simulink model "Module1QuizModel"  (R2026a)
settings: Solver=VariableStepAuto  StopTime=7200
libraries: fl_lib x4, batt_lib x2, simulink x2, nesl_utility x1
settings Model: Creator=sturton  LastModifiedBy=User
settings SimscapeCC: SimscapeNominalValues="[{\"value\":\"1\",\"unit\":\"A\"},{\"value\":\"1\",\"unit\":\"bar\"},{\"value\":\"1\",\"unit\":\"cm^2\"},{\"value\":\"1\",\"unit\":\"cm^3/s\"},{\"value\":\"1\",\"unit\":\"kJ/kg\"},{\"value\":\"1\",\"unit\":\"kW\"},{\"value\":\"1\",\"unit\":\"l\"},{\"value\":\"1\",\"unit\":\"N\"},{\"value\":\"1\",\"unit\":\"N*m\"},{\"value\":\"1\",\"unit\":\"V\"}]"  SimscapeLogType=none  SimscapeLogDataHistory=5000.0

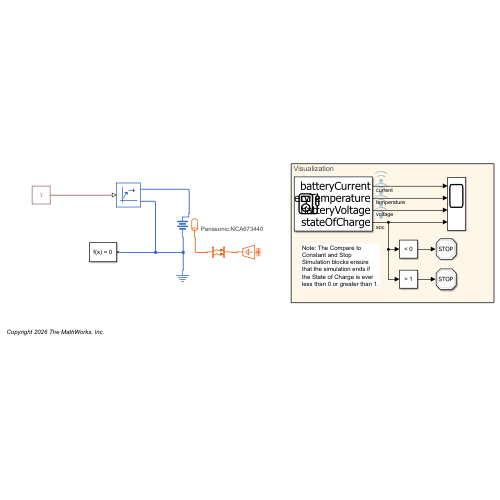
[thumbnail: Simulink's stored preview of the top-level diagram]
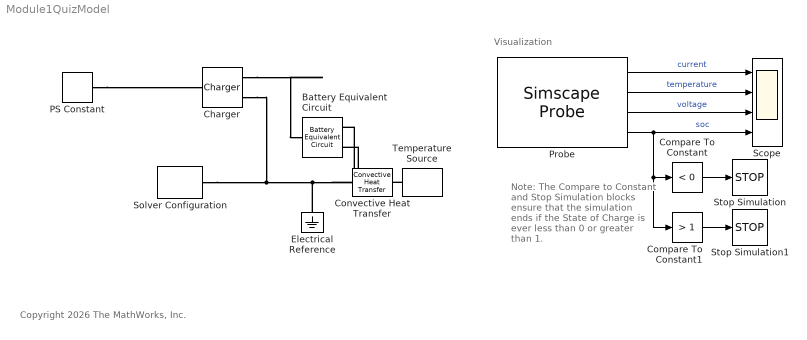
== system Module1QuizModel ==
  note: Note: The Compare to Constant and Stop Simulation blocks ensure that the simulation ends if the State of Charge is ever less than 0 or greater than 1.
  note: Visualization
  note: Copyright 2026 The MathWorks, Inc.
  Battery Equivalent Circuit : batt_lib/Cells/Battery Equivalent Circuit  PartSpecification="{\"CollectionId\":\"MW.SimscapeBattery\",\"CollectionVersion\":\"1.0.0\",\"DatasetId\":\"Panasonic|NCA673440|simscape.battery.batteryEquivalentCircuit\",\"DisplayName\":\"Panasonic:NCA673440\"}"  BatteryCapacity=1.236 % Datasheet derived hr*A  ThermalModel=simscape.battery.enum.cells.BatteryThermalModel.LumpedThermalMass  ExtrapolationMethod=simscape.enum.extrapolation.linear  SOCBreakpoints=[0 0.01 0.02 0.03 0.04 0.05 0.06 0.07 0.08 0.09 0.1 0.11 0.12 0.13 0.14 0.15 0.16 0.17 0.18 0.19 0.2 0.21 0.22 0.23 0.24 0.25 0.26 0.27 0.28 0.29 0.3 0.31 0.32 0.33 0.34 0.35 0.36 0.37 0.38 0.39 0.4 0.41 0.42 0.43 0.44 0.45 0.46 0.47 0.48 0.49 0.5 0.51 0.52 0.53 0.54 0.55 0.56 0.57 0.58 0.59 0.6 0.61 0.62 0.63 0.64 0.65 0.66 0.67 0.68 0.69 0.7 0.71 0.72 0.73 0.74 0.75 0.76 0.77 0.78 0.79 0.8 0.81 0.82 0.83 0.84 0.85 0.86 0.87 0.88 0.89 0.9 0.91 0.92 0.93 0.94 0.95 0.96 0.97 0.98 0.99 1] % Datasheet derived  TemperatureBreakpoints=[-20 -10 0 25 40] % Datasheet derived degC  OpenCircuitVoltage=[2.81282 2.92952 3.02616 3.09882 3.15595 3.19736 3.23687 3.2696 3.29224 3.3165 3.33606 3.35376 3.37201 3.38673 3.40034 3.412 3.42329 3.4339 3.44451 3.45615 3.466 3.4726 3.47919 3.48579 3.49239 3.49904 3.50604 3.51305 3.52005 3.52703 3.53325 3.53921 3.54518 3.55115 3.55712 3.56323 3.5696 3.57596 3.58233 3.58876 3.59531 3.60186 3.60839 3.61485 3.62133 3.62799 3.63464 3.64129 3.64862 3.65637 3.6643 3.67241 3.68051 3.68861 3.69647 3.70506 3.71368 3.7223 3.731 3.74039 3.74966 3.75893 3.76819 3.77737 3.78644 3.79552 3.80425 3.81234 3.82043 3.82859 3.83695 3.84539 3.85383 3.86227 3.87071 3.87916 3.8876 3.89604 3.90651 3.91746 3.92861 3.94006 3.95152 3.96297 3.97442 3.98588 3.99733 4.0089 4.02025 4.03129 4.04215 4.0529 4.06366 4.07442 4.0852 4.09635 4.1089 4.1233 4.13483 4.15326 4.13871] % Datasheet derived V  OpenCircuitVoltageThermal=[2.81282 2.81282 2.81282 2.81282 2.81282;2.92952 2.92952 2.92952 2.92952 2.92952;3.02616 3.02616 3.02616 3.02616 3.02616;3.09882 3.09882 3.09882 3.09882 3.09882;3.15595 3.15595 3.15595 3.15595 3.15595;3.19736 3.19736 3.19736 3.19736 3.19736;3.23687 3.23687 3.23687 3.23687 3.23687;3.2696 3.2696 3.2696 3.2696 3.2696;3.29224 3.29224 3.29224 3.29224 3.29224;3.3165 3.3165 3.3165 3.3165 3.3165;3.33606 3.33606 3.33606 3.33606 3.33606;3.35376 3.35376 3.35376 3.35376 3.35376;3.37201 3.37201 3.37201 3.37201 3.37201;3.38673 3.38673 3.38673 3.38673 3.38673;3.40034 3.40034 3.40034 3.40034 3.40034;3.412 3.412 3.412 3.412 3.412;3.42329 3.42329 3.42329 3.42329 3.42329;3.4339 3.4339 3.4339 3.4339 3.4339;3.44451 3.44451 3.44451 3.44451 3.44451;3.45615 3.45615 3.45615 3.45615 3.45615;3.466 3.466 3.466 3.466 3.466;3.4726 3.4726 3.4726 3.4726 3.4726;3.47919 3.47919 3.47919 3.47919 3.47919;3.48579 3.48579 3.48579 3.48579 3.48579;3.49239 3.49239 3.49239 3.49239 3.49239;3.49904 3.49904 3.49904 3.49904 3.49904;3.50604 3.50604 3.50604 3.50604 3.50604;3.51305 3.51305 3.51305 3.51305 3.51305;3.52005 3.52005 3.52005 3.52005 3.52005;3.52703 3.52703 3.52703 3.52703 3.52703;3.53325 3.53325 3.53325 3.53325 3.53325;3.53921 3.53921 3.53921 3.53921 3.53921;3.54518 3.54518 3.54518 3.54518 3.54518;3.55115 3.55115 3.55115 3.55115 3.55115;3.55712 3.55712 3.55712 3.55712 3.55712;3.56323 3.56323 3.56323 3.56323 3.56323;3.5696 3.5696 3.5696 3.5696 3.5696;3.57596 3.57596 3.57596 3.57596 3.57596;3.58233 3.58233 3.58233 3.58233 3.58233;3.58876 3.58876 3.58876 3.58876 3.58876;3.59531 3.59531 3.59531 3.59531 3.59531;3.60186 3.60186 3.60186 3.60186 3.60186;3.60839 3.60839 3.60839 3.60839 3.60839;3.61485 3.61485 3.61485 3.61485 3.61485;3.62133 3.62133 3.62133 3.62133 3.62133;3.62799 3.62799 3.62799 3.62799 3.62799;3.63464 3.63464 3.63464 3.63464 3.63464;3.64129 3.64129 3.64129 3.64129 3.64129;3.64862 3.64862 3.64862 3.64862 3.64862;3.65637 3.65637 3.65637 3.65637 3.65637;3.6643 3.6643 3.6643 3.6643 3.6643;3.67241 3.67241 3.67241 3.67241 3.67241;3.68051 3.68051 3.68051 3.68051 3.68051;3.68861 3.68861 3.68861 3.68861 3.68861;3.69647 3.69647 3.69647 3.69647 3.69647;3.70506 3.70506 3.70506 3.70506 3.70506;3.71368 3.71368 3.71368 3.71368 3.71368;3.7223 3.7223 3.7223 3.7223 3.7223;3.731 3.731 3.731 3.731 3.731;3.74039 3.74039 3.74039 3.74039 3.74039;3.74966 3.74966 3.74966 3.74966 3.74966;3.75893 3.75893 3.75893 3.75893 3.75893;3.76819 3.76819 3.76819 3.76819 3.76819;3.77737 3.77737 3.77737 3.77737 3.77737;3.78644 3.78644 3.78644 3.78644 3.78644;3.79552 3.79552 3.79552 3.79552 3.79552;3.80425 3.80425 3.80425 3.80425 3.80425;3.81234 3.81234 3.81234 3.81234 3.81234;3.82043 3.82043 3.82043 3.82043 3.82043;3.82859 3.82859 3.82859 3.82859 3.82859;3.83695 3.83695 3.83695 3.83695 3.83695;3.84539 3.84539 3.84539 3.84539 3.84539;3.85383 3.85383 3.85383 3.85383 3.85383;3.86227 3.86227 3.86227 3.86227 3.86227;3.87071 3.87071 3.87071 3.87071 3.87071;3.87916 3.87916 3.87916 3.87916 3.87916;3.8876 3.8876 3.8876 3.8876 3.8876;3.89604 3.89604 3.89604 3.89604 3.89604;3.90651 3.90651 3.90651 3.90651 3.90651;3.91746 3.91746 3.91746 3.91746 3.91746;3.92861 3.92861 3.92861 3.92861 3.92861;3.94006 3.94006 3.94006 3.94006 3.94006;3.95152 3.95152 3.95152 3.95152 3.95152;3.96297 3.96297 3.96297 3.96297 3.96297;3.97442 3.97442 3.97442 3.97442 3.97442;3.98588 3.98588 3.98588 3.98588 3.98588;3.99733 3.99733 3.99733 3.99733 3.99733;4.0089 4.0089 4.0089 4.0089 4.0089;4.02025 4.02025 4.02025 4.02025 4.02025;4.03129 4.03129 4.03129 4.03129 4.03129;4.04215 4.04215 4.04215 4.04215 4.04215;4.0529 4.0529 4.0529 4.0529 4.0529;4.06366 4.06366 4.06366 4.06366 4.06366;4.07442 4.07442 4.07442 4.07442 4.07442;4.0852 4.0852 4.0852 4.0852 4.0852;4.09635 4.09635 4.09635 4.09635 4.09635;4.1089 4.1089 4.1089 4.1089 4.1089;4.1233 4.1233 4.1233 4.1233 4.1233;4.13483 4.13483 4.13483 4.13483 4.13483;4.15326 4.15326 4.15326 4.15326 4.15326;4.13871 4.13871 4.13871 4.13871 4.13871] % Datasheet derived V  VoltageRange=[2.475 Inf] % Datasheet derived V  HysteresisModel=simscape.battery.enum.cells.HysteresisModel.none  MaximumHysteresisVoltage=[0, 0, 0, 0, 0, 0, 0] % Parameter not set V  InstantaneousHysteresisVoltage=[0, 0, 0, 0, 0, 0, 0] % Parameter not set V  HysteresisRate=0.1 % Parameter not set  MaximumHysteresisVoltageThermal=[0, 0, 0; 0, 0, 0; 0, 0, 0; 0, 0, 0; 0, 0, 0; 0, 0, 0; 0, 0, 0] % Parameter not set V  InstantaneousHysteresisVoltageThermal=[0, 0, 0; 0, 0, 0; 0, 0, 0; 0, 0, 0; 0, 0, 0; 0, 0, 0; 0, 0, 0] % Parameter not set V  HysteresisRateThermal=0.1 % Parameter not set  ResistanceSOCBreakpoints=[0 0.01 0.02 0.03 0.04 0.05 0.06 0.07 0.08 0.09 0.1 0.11 0.12 0.13 0.14 0.15 0.16 0.17 0.18 0.19 0.2 0.21 0.22 0.23 0.24 0.25 0.26 0.27 0.28 0.29 0.3 0.31 0.32 0.33 0.34 0.35 0.36 0.37 0.38 0.39 0.4 0.41 0.42 0.43 0.44 0.45 0.46 0.47 0.48 0.49 0.5 0.51 0.52 0.53 0.54 0.55 0.56 0.57 0.58 0.59 0.6 0.61 0.62 0.63 0.64 0.65 0.66 0.67 0.68 0.69 0.7 0.71 0.72 0.73 0.74 0.75 0.76 0.77 0.78 0.79 0.8 0.81 0.82 0.83 0.84 0.85 0.86 0.87 0.88 0.89 0.9 0.91 0.92 0.93 0.94 0.95 0.96 0.97 0.98 0.99 1] % Datasheet derived  ResistanceTemperatureBreakpoints=[-20 -10 0 25 40] % Datasheet derived degC  ResistanceCurrentBreakpoints=[-1, 0, 1] % Parameter not set A  CurrentDependence=simscape.battery.enum.cells.CurrentDependence.Disabled  R0=[0.1195 0.14734 0.16452 0.17097 0.16988 0.16446 0.16485 0.16445 0.16084 0.15998 0.15922 0.15784 0.1574 0.1565 0.15518 0.15284 0.15055 0.14837 0.14619 0.14574 0.14532 0.1435 0.14169 0.13987 0.13805 0.13632 0.13519 0.13407 0.13294 0.1318 0.13054 0.1292 0.12787 0.12654 0.1252 0.12412 0.12346 0.1228 0.12215 0.12145 0.12073 0.12001 0.11928 0.11852 0.11781 0.11738 0.11695 0.11652 0.11644 0.1166 0.11673 0.11683 0.11693 0.11703 0.11671 0.1163 0.11591 0.11551 0.11516 0.11517 0.11521 0.11524 0.11527 0.11514 0.11486 0.11457 0.11414 0.11345 0.11275 0.11209 0.11172 0.1115 0.11127 0.11105 0.11082 0.1106 0.11037 0.11014 0.11063 0.11131 0.11219 0.1136 0.115 0.11641 0.11781 0.11921 0.12062 0.12211 0.12357 0.1249 0.12592 0.12677 0.12761 0.12845 0.12929 0.13023 0.13186 0.13449 0.1303 0.12272 0.05007] % Datasheet derived Ohm  R0I=[.0117, .0085, .009; .011, .0085, .009; .0114, .0087, .0092; .0107, .0082, .0088; .0107, .0083, .0091; .0113, .0085, .0089; .0116, .0085, .0089] % Parameter not set Ohm  R0Thermal=[0.91507 0.64886 0.76779 0.1195 0.07217;0.91507 0.9802 1.05708 0.14734 0.05983;0.91507 0.95979 1.01635 0.16452 0.04254;0.91507 0.93938 0.97562 0.17097 0.05718;0.91507 0.91897 0.93489 0.16988 0.06137;0.91507 0.89855 0.89416 0.16446 0.07086;0.91507 0.87814 0.85343 0.16485 0.07883;0.91507 0.85773 0.8127 0.16445 0.09222;0.91507 0.83732 0.77197 0.16084 0.09721;0.91507 0.81691 0.73124 0.15998 0.10355;0.91507 0.7965 0.69051 0.15922 0.10881;0.91507 0.77608 0.64978 0.15784 0.11252;0.91507 0.75567 0.60905 0.1574 0.11668;0.90135 0.73526 0.56832 0.1565 0.11813;0.88763 0.71485 0.52759 0.15518 0.11951;0.87392 0.69444 0.48527 0.15284 0.11926;0.8602 0.67403 0.45861 0.15055 0.1187;0.84648 0.65361 0.43204 0.14837 0.11758;0.83276 0.6332 0.41039 0.14619 0.11645;0.81904 0.61279 0.39684 0.14574 0.11867;0.80533 0.59091 0.38181 0.14532 0.11977;0.79161 0.56633 0.36407 0.1435 0.11817;0.77789 0.54174 0.3476 0.14169 0.11656;0.76417 0.51715 0.33715 0.13987 0.11495;0.75045 0.49671 0.32669 0.13805 0.11335;0.73674 0.48301 0.31628 0.13632 0.11191;0.72302 0.4696 0.30882 0.13519 0.11096;0.7093 0.4562 0.30303 0.13407 0.11001;0.69558 0.4428 0.29723 0.13294 0.10905;0.68186 0.42937 0.29142 0.1318 0.10807;0.66815 0.41843 0.28497 0.13054 0.10646;0.65423 0.41062 0.28038 0.1292 0.10465;0.64032 0.40281 0.27663 0.12787 0.10283;0.6264 0.395 0.27288 0.12654 0.10101;0.61249 0.38719 0.26913 0.1252 0.09919;0.5987 0.3795 0.2655 0.12412 0.09826;0.58512 0.37203 0.26209 0.12346 0.0977;0.57153 0.36581 0.25916 0.1228 0.09714;0.55932 0.36186 0.25623 0.12215 0.09658;0.55177 0.35796 0.25335 0.12145 0.09608;0.54432 0.35417 0.25057 0.12073 0.09567;0.53687 0.35037 0.24779 0.12001 0.09527;0.5294 0.34656 0.24499 0.11928 0.09484;0.52187 0.34269 0.24214 0.11852 0.09436;0.51437 0.33884 0.2393 0.11781 0.0939;0.507 0.33512 0.23677 0.11738 0.09322;0.50125 0.33141 0.23475 0.11695 0.0919;0.49572 0.32777 0.23274 0.11652 0.09057;0.49076 0.3247 0.23129 0.11644 0.08981;0.48615 0.32199 0.23019 0.1166 0.0894;0.48169 0.31942 0.22925 0.11673 0.08914;0.47738 0.317 0.22844 0.11683 0.08902;0.47306 0.31457 0.22764 0.11693 0.0889;0.46874 0.31215 0.22683 0.11703 0.08879;0.46462 0.30952 0.22582 0.11671 0.08846;0.46133 0.3075 0.22542 0.1163 0.08795;0.45807 0.30632 0.22505 0.11591 0.08735;0.4548 0.3054 0.22468 0.11551 0.08676;0.4516 0.30454 0.22428 0.11516 0.08623;0.44899 0.30426 0.22355 0.11517 0.08628;0.44626 0.30388 0.22271 0.11521 0.08622;0.44354 0.3035 0.22188 0.11524 0.08617;0.44082 0.30312 0.22104 0.11527 0.08611;0.43851 0.30265 0.22013 0.11514 0.08598;0.4385 0.30212 0.21913 0.11486 0.08576;0.4385 0.30158 0.21814 0.11457 0.08555;0.4382 0.30094 0.21686 0.11414 0.08505;0.43737 0.30006 0.21504 0.11345 0.08401;0.43654 0.29918 0.21322 0.11275 0.08322;0.43576 0.29836 0.21146 0.11209 0.08264;0.43516 0.2977 0.21187 0.11172 0.08223;0.43462 0.29712 0.21246 0.1115 0.08189;0.43513 0.29653 0.21305 0.11127 0.08154;0.43636 0.29594 0.21363 0.11105 0.0812;0.43759 0.29536 0.21422 0.11082 0.08086;0.43882 0.29583 0.21481 0.1106 0.08051;0.44004 0.29808 0.21539 0.11037 0.08017;0.44127 0.30032 0.21598 0.11014 0.07983;0.44419 0.30425 0.21826 0.11063 0.08056;0.4475 0.30858 0.22093 0.11131 0.08006;0.45099 0.31308 0.22434 0.11219 0.07972;0.45473 0.31784 0.22962 0.1136 0.07964;0.46234 0.32313 0.2349 0.115 0.07955;0.47176 0.33193 0.24018 0.11641 0.07947;0.48119 0.34073 0.24546 0.11781 0.07938;0.49061 0.34953 0.25074 0.11921 0.0793;0.50004 0.35833 0.25602 0.12062 0.07955;0.50956 0.36723 0.2645 0.12211 0.0805;0.5224 0.37673 0.27312 0.12357 0.08126;0.54766 0.39209 0.28148 0.1249 0.08177;0.57277 0.4073 0.2897 0.12592 0.08213;0.60249 0.42242 0.29782 0.12677 0.0824;0.63849 0.43753 0.30705 0.12761 0.08267;0.67449 0.45424 0.31684 0.12845 0.08292;0.71052 0.47435 0.32664 0.12929 0.08317;0.7543 0.49476 0.33675 0.13023 0.08373;0.79949 0.51481 0.34571 0.13186 0.08544;0.84623 0.53557 0.355 0.13449 0.08871;0.86284 0.54572 0.36189 0.1303 0.08803;0.87986 0.53749 0.35636 0.12272 0.08074;0.76995 0.47785 0.31756 0.05007 0.04597] % Datasheet derived Ohm  R0ThermalI=repmat([.0117, .0085, .009; .011, .0085, .009; .0114, .0087, .0092; .0107, .0082, .0088; .0107, .0083, .0091; .0113, .0085, .0089; .0116, .0085, .0089], 1, 1, 3) % Parameter not set Ohm  DischargeR0=[.0085, .0085, .0087, .0082, .0083, .0085, .0085] % Parameter not set Ohm  ChargeR0=[.0085, .0085, .0087, .0082, .0083, .0085, .0085] % Parameter not set Ohm  ChargeR0Thermal=[.0117, .0085, .009; .011, .0085, .009; .0114, .0087, .0092; .0107, .0082, .0088; .0107, .0083, .0091; .0113, .0085, .0089; .0116, .0085, .0089] % Parameter not set Ohm  DischargeR0Thermal=[.0117, .0085, .009; .011, .0085, .009; .0114, .0087, .0092; .0107, .0082, .0088; .0107, .0083, .0091; .0113, .0085, .0089; .0116, .0085, .0089] % Parameter not set Ohm  RCPairs=simscape.battery.enum.cells.RCPairs.noDynamics  R1=[.0029, .0024, .0026, .0016, .0023, .0018, .0017] % Parameter not set Ohm  Tau1=[36, 45, 105, 29, 77, 33, 39] % Parameter not set s  R2=[.0029, .0024, .0026, .0016, .0023, .0018, .0017] % Parameter not set Ohm  Tau2=[36, 45, 105, 29, 77, 33, 39] % Parameter not set s  R3=[.0029, .0024, .0026, .0016, .0023, .0018, .0017] % Parameter not set Ohm  Tau3=[36, 45, 105, 29, 77, 33, 39] % Parameter not set s  R1I=[.0109, .0029, .0013; .0069, .0024, .0012; .0047, .0026, .0013; .0034, .0016, .001; .0033, .0023, .0014; .0033, .0018, .0011; .0028, .0017, .0011] % Parameter not set Ohm  Tau1I=[20, 36, 39; 31, 45, 39; 109, 105, 61; 36, 29, 26; 59, 77, 67; 40, 33, 29; 25, 39, 33] % Parameter not set s  R2I=[.0109, .0029, .0013; .0069, .0024, .0012; .0047, .0026, .0013; .0034, .0016, .001; .0033, .0023, .0014; .0033, .0018, .0011; .0028, .0017, .0011] % Parameter not set Ohm  Tau2I=[20, 36, 39; 31, 45, 39; 109, 105, 61; 36, 29, 26; 59, 77, 67; 40, 33, 29; 25, 39, 33] % Parameter not set s  R3I=[.0109, .0029, .0013; .0069, .0024, .0012; .0047, .0026, .0013; .0034, .0016, .001; .0033, .0023, .0014; .0033, .0018, .0011; .0028, .0017, .0011] % Parameter not set Ohm  Tau3I=[20, 36, 39; 31, 45, 39; 109, 105, 61; 36, 29, 26; 59, 77, 67; 40, 33, 29; 25, 39, 33] % Parameter not set s  DischargeR1=[.0029, .0024, .0026, .0016, .0023, .0018, .0017] % Parameter not set Ohm  DischargeTau1=[36, 45, 105, 29, 77, 33, 39] % Parameter not set s  ChargeR1=[.0029, .0024, .0026, .0016, .0023, .0018, .0017] % Parameter not set Ohm  ChargeTau1=[36, 45, 105, 29, 77, 33, 39] % Parameter not set s  DischargeR2=[.0029, .0024, .0026, .0016, .0023, .0018, .0017] % Parameter not set Ohm  DischargeTau2=[36, 45, 105, 29, 77, 33, 39] % Parameter not set s  ChargeR2=[.0029, .0024, .0026, .0016, .0023, .0018, .0017] % Parameter not set Ohm  ChargeTau2=[36, 45, 105, 29, 77, 33, 39] % Parameter not set s  DischargeR3=[.0029, .0024, .0026, .0016, .0023, .0018, .0017] % Parameter not set Ohm  DischargeTau3=[36, 45, 105, 29, 77, 33, 39] % Parameter not set s  ChargeR3=[.0029, .0024, .0026, .0016, .0023, .0018, .0017] % Parameter not set Ohm  ChargeTau3=[36, 45, 105, 29, 77, 33, 39] % Parameter not set s  R1Thermal=[.0109, .0029, .0013; .0069, .0024, .0012; .0047, .0026, .0013; .0034, .0016, .001; .0033, .0023, .0014; .0033, .0018, .0011; .0028, .0017, .0011] % Parameter not set Ohm  Tau1Thermal=[20, 36, 39; 31, 45, 39; 109, 105, 61; 36, 29, 26; 59, 77, 67; 40, 33, 29; 25, 39, 33] % Parameter not set s  R2Thermal=[.0109, .0029, .0013; .0069, .0024, .0012; .0047, .0026, .0013; .0034, .0016, .001; .0033, .0023, .0014; .0033, .0018, .0011; .0028, .0017, .0011] % Parameter not set Ohm  Tau2Thermal=[20, 36, 39; 31, 45, 39; 109, 105, 61; 36, 29, 26; 59, 77, 67; 40, 33, 29; 25, 39, 33] % Parameter not set s  R3Thermal=[.0109, .0029, .0013; .0069, .0024, .0012; .0047, .0026, .0013; .0034, .0016, .001; .0033, .0023, .0014; .0033, .0018, .0011; .0028, .0017, .0011] % Parameter not set Ohm  Tau3Thermal=[20, 36, 39; 31, 45, 39; 109, 105, 61; 36, 29, 26; 59, 77, 67; 40, 33, 29; 25, 39, 33] % Parameter not set s  R1ThermalI=repmat([.0109, .0029, .0013; .0069, .0024, .0012; .0047, .0026, .0013; .0034, .0016, .001; .0033, .0023, .0014; .0033, .0018, .0011; .0028, .0017, .0011], 1, 1, 3) % Parameter not set Ohm  Tau1ThermalI=repmat([20, 36, 39; 31, 45, 39; 109, 105, 61; 36, 29, 26; 59, 77, 67; 40, 33, 29; 25, 39, 33], 1, 1, 3) % Parameter not set s  R2ThermalI=repmat([.0109, .0029, .0013; .0069, .0024, .0012; .0047, .0026, .0013; .0034, .0016, .001; .0033, .0023, .0014; .0033, .0018, .0011; .0028, .0017, .0011], 1, 1, 3) % Parameter not set Ohm  Tau2ThermalI=repmat([20, 36, 39; 31, 45, 39; 109, 105, 61; 36, 29, 26; 59, 77, 67; 40, 33, 29; 25, 39, 33], 1, 1, 3) % Parameter not set s  R3ThermalI=repmat([.0109, .0029, .0013; .0069, .0024, .0012; .0047, .0026, .0013; .0034, .0016, .001; .0033, .0023, .0014; .0033, .0018, .0011; .0028, .0017, .0011], 1, 1, 3) % Parameter not set Ohm  Tau3ThermalI=repmat([20, 36, 39; 31, 45, 39; 109, 105, 61; 36, 29, 26; 59, 77, 67; 40, 33, 29; 25, 39, 33], 1, 1, 3) % Parameter not set s  DischargeR1Thermal=[.0109, .0029, .0013; .0069, .0024, .0012; .0047, .0026, .0013; .0034, .0016, .001; .0033, .0023, .0014; .0033, .0018, .0011; .0028, .0017, .0011] % Parameter not set Ohm  DischargeTau1Thermal=[20, 36, 39; 31, 45, 39; 109, 105, 61; 36, 29, 26; 59, 77, 67; 40, 33, 29; 25, 39, 33] % Parameter not set s  ChargeR1Thermal=[.0109, .0029, .0013; .0069, .0024, .0012; .0047, .0026, .0013; .0034, .0016, .001; .0033, .0023, .0014; .0033, .0018, .0011; .0028, .0017, .0011] % Parameter not set Ohm  ChargeTau1Thermal=[20, 36, 39; 31, 45, 39; 109, 105, 61; 36, 29, 26; 59, 77, 67; 40, 33, 29; 25, 39, 33] % Parameter not set s  DischargeR2Thermal=[.0109, .0029, .0013; .0069, .0024, .0012; .0047, .0026, .0013; .0034, .0016, .001; .0033, .0023, .0014; .0033, .0018, .0011; .0028, .0017, .0011] % Parameter not set Ohm  DischargeTau2Thermal=[20, 36, 39; 31, 45, 39; 109, 105, 61; 36, 29, 26; 59, 77, 67; 40, 33, 29; 25, 39, 33] % Parameter not set s  ChargeR2Thermal=[.0109, .0029, .0013; .0069, .0024, .0012; .0047, .0026, .0013; .0034, .0016, .001; .0033, .0023, .0014; .0033, .0018, .0011; .0028, .0017, .0011] % Parameter not set Ohm  ChargeTau2Thermal=[20, 36, 39; 31, 45, 39; 109, 105, 61; 36, 29, 26; 59, 77, 67; 40, 33, 29; 25, 39, 33] % Parameter not set s  DischargeR3Thermal=[.0109, .0029, .0013; .0069, .0024, .0012; .0047, .0026, .0013; .0034, .0016, .001; .0033, .0023, .0014; .0033, .0018, .0011; .0028, .0017, .0011] % Parameter not set Ohm  DischargeTau3Thermal=[20, 36, 39; 31, 45, 39; 109, 105, 61; 36, 29, 26; 59, 77, 67; 40, 33, 29; 25, 39, 33] % Parameter not set s  ChargeR3Thermal=[.0109, .0029, .0013; .0069, .0024, .0012; .0047, .0026, .0013; .0034, .0016, .001; .0033, .0023, .0014; .0033, .0018, .0011; .0028, .0017, .0011] % Parameter not set Ohm  ChargeTau3Thermal=[20, 36, 39; 31, 45, 39; 109, 105, 61; 36, 29, 26; 59, 77, 67; 40, 33, 29; 25, 39, 33] % Parameter not set s  SelfDischargeResistor=simscape.battery.enum.cells.BatteryEnable.Disabled  SelfDischargeR=7e3 % Parameter not set Ohm  SelfDischargeRThermal=[8000, 7000, 6000] % Parameter not set Ohm  CyclingAgingMethod=simscape.battery.enum.cells.CyclingAgingMethod.tableN  CycleCalculationMethod=simscape.battery.enum.cells.CycleCalculationMethod.EquivalentCycles  NumDisCycles=100 % Parameter not set  OCVChange=0 % Parameter not set  R0Change=0 % Parameter not set  CapacityChange=0 % Parameter not set  SelfDischargeRChange=0 % Parameter not set  R1Change=0 % Parameter not set  R2Change=0 % Parameter not set  R3Change=0 % Parameter not set  NumDisCyclesBreakpoints=[0 6 11 16 21 26 31 36 41 46 51 56 61 66 71 76 81 86 91 96 101 106 111 116 121 126 131 136 141 146 151 156 161 166 171 176 181 186 191 196 201 206 211 216 221 226 231 236 241 246 251 256 261 266 271 276 281 286 291 296 301 306 311 316 321 326 331 336 341 346 351 356 361 366 371 376 381 386 391 396 401 406 411 416 421 426 431 436 441 446 451 456 461 466 471 476 481 486 491 496] % Datasheet derived  AgingTemperatureBreakpoints=[298.15, 323.15] % Parameter not set K  AgingCurrentBreakpoints=[-.1, -.5, -5] % Parameter not set A  OCVChangeVec=[0 0.1247 0.2494 0.323 0.165 0.0602 -0.0255 -0.1046 -0.1582 -0.2117 -0.2653 -0.3199 -0.3772 -0.4475 -0.5179 -0.5882 -0.6586 -0.7278 -0.7891 -0.8504 -0.9116 -0.9729 -1.0312 -1.0803 -1.1294 -1.1785 -1.2276 -1.2768 -1.3248 -1.3723 -1.4198 -1.4673 -1.5148 -1.5622 -1.6096 -1.6569 -1.7085 -1.7602 -1.812 -1.8637 -1.9155 -1.9672 -2.019 -2.0707 -2.1225 -2.1742 -2.226 -2.2777 -2.3295 -2.3817 -2.4275 -2.47 -2.5126 -2.5551 -2.5976 -2.6408 -2.6841 -2.7273 -2.7705 -2.8137 -2.8569 -2.9012 -2.9456 -2.99 -3.0344 -3.0788 -3.1232 -3.1669 -3.2021 -3.2373 -3.2726 -3.3078 -3.343 -3.3782 -3.4135 -3.4484 -3.4833 -3.5182 -3.5531 -3.5879 -3.6228 -3.6577 -3.7072 -3.7621 -3.817 -3.872 -3.9269 -3.9818 -4.0367 -4.0916 -4.1465 -4.1989 -4.2489 -4.2989 -4.3489 -4.3989 -4.4489 -4.4989 -4.5489 -4.5989] % Datasheet derived  OCVChangeThermal=[0, 0; 0, 0; 0, 0; 0, 0] % Parameter not set  R0ChangeVec=[0 0 0 0 0 0 0 0 0 0 0 0 0 0 0 0 0 0 0 0 0 0 0 0 0 0 0 0 0 0 0 0 0 0 0 0 0 0 0 0 0 0 0 0 0 0 0 0 0 0 0 0 0 0 0 0 0 0 0 0 0 0 0 0 0 0 0 0 0 0 0 0 0 0 0 0 0 0 0 0 0 0 0 0 0 0 0 0 0 0 0 0 0 0 0 0 0 0 0 0] % Parameter assumed  R0ChangeThermal=[0, 0; 0, 0; 0, 0; 0, 0] % Parameter not set  R0ChangeThermalI=repmat(0, 4, 2, 3) % Parameter not set  R0CyclingChangeInitialTarget=0 % Parameter not set  CapacityChangeVec=[0 -0.355 -0.709 -1.064 -1.419 -1.654 -1.847 -2.039 -2.231 -2.424 -2.616 -2.812 -3.014 -3.216 -3.419 -3.621 -3.823 -4.025 -4.227 -4.429 -4.631 -4.833 -5.029 -5.211 -5.394 -5.576 -5.758 -5.94 -6.123 -6.305 -6.487 -6.669 -6.852 -7.034 -7.216 -7.398 -7.597 -7.796 -7.995 -8.194 -8.393 -8.592 -8.791 -8.991 -9.19 -9.389 -9.588 -9.787 -9.986 -10.185 -10.36 -10.522 -10.684 -10.846 -11.008 -11.17 -11.332 -11.494 -11.656 -11.818 -11.98 -12.142 -12.304 -12.466 -12.628 -12.79 -12.952 -13.109 -13.235 -13.361 -13.487 -13.613 -13.739 -13.865 -13.991 -14.117 -14.243 -14.369 -14.495 -14.622 -14.748 -14.874 -15.053 -15.251 -15.449 -15.648 -15.846 -16.045 -16.243 -16.441 -16.64 -16.829 -17.01 -17.191 -17.371 -17.552 -17.733 -17.913 -18.094 -18.275] % Datasheet derived  CapacityChangeThermal=[0, 0; 0, 0; 0, 0; 0, 0] % Parameter not set  CapacityChangeThermalI=repmat(0, 4, 2, 3) % Parameter not set  CapacityCyclingChangeInitialTarget=0 % Parameter not set  SelfDischargeRChangeVec=[0, 0, 0, 0] % Parameter not set  SelfDischargeRChangeThermal=[0, 0; 0, 0; 0, 0; 0, 0] % Parameter not set  SelfDischargeRChangeThermalI=repmat(0, 4, 2, 3) % Parameter not set  SelfDischargeRCyclingChangeInitialTarget=0 % Parameter not set  R1ChangeVec=[0, 0, 0, 0] % Parameter not set  R1ChangeThermal=[0, 0; 0, 0; 0, 0; 0, 0] % Parameter not set  R1ChangeThermalI=repmat(0, 4, 2, 3) % Parameter not set  R1CyclingChangeInitialTarget=0 % Parameter not set  R2ChangeVec=[0, 0, 0, 0] % Parameter not set  R2ChangeThermal=[0, 0; 0, 0; 0, 0; 0, 0] % Parameter not set  R2ChangeThermalI=repmat(0, 4, 2, 3) % Parameter not set  R2CyclingChangeInitialTarget=0 % Parameter not set  R3ChangeVec=[0, 0, 0, 0] % Parameter not set  R3ChangeThermal=[0, 0; 0, 0; 0, 0; 0, 0] % Parameter not set  R3ChangeThermalI=repmat(0, 4, 2, 3) % Parameter not set  R3CyclingChangeInitialTarget=0 % Parameter not set  CalendarAgeResistance=simscape.battery.enum.cells.BatteryEnable.Disabled  CalendarAgeCapacity=simscape.battery.enum.cells.BatteryEnable.Disabled  CalendarAgingMethod=simscape.battery.enum.cells.CalendarAgingMethod.equation  StorageVariable=simscape.battery.enum.cells.StorageVariable.OCV  OCVDuringStorage=0.9 % Parameter not set  SOCDuringStorage=0.6 % Parameter not set  StorageTimeIntervals=[0] % Parameter not set d  StorageTemperatures=[273] % Parameter not set K  ResistanceScalingOCV=2.2134e6 % Parameter not set  ResistanceScalingOCVOffset=1.632e6 % Parameter not set  ResistanceExponentialIncrease=0.515833569 % Parameter not set V  ResistanceTimeExponent=0.75 % Parameter not set  ResistanceAgeTemperatureBreakpoints=[273.15, 298.15, 323.15] % Parameter not set K  ResistanceAgeTimeBreakpoints=[0, 90, 180, 270] % Parameter not set d  PercentResistanceChange=[0, 0, 0] % Parameter not set  ResistanceTimeBreakpoints=100 % Parameter not set d  PercentResistanceChangeThermal=[0, 0, 0; 0, 0, 0; 0, 0, 0; 0, 0, 0] % Parameter not set  CapacityScalingOCV=1.5097e07 % Parameter not set  CapacityScalingOCVOffset=8.3625e06 % Parameter not set  CapacityExponentialIncrease=0.6011 % Parameter not set V  CapacityTimeExponent=0.75 % Parameter not set  CapacityAgeTemperatureBreakpoints=[273.15, 298.15, 323.15] % Parameter not set K  CapacityAgeTimeBreakpoints=[0, 90, 180, 270] % Parameter not set d  PercentCapacityChange=[0, 0, 0] % Parameter not set  CapacityTimeBreakpoints=100 % Parameter not set d  PercentCapacityChangeThermal=[0, 0, 0; 0, 0, 0; 0, 0, 0; 0, 0, 0] % Parameter not set  SimulationTemperature=298.15 % Parameter not set K  BatteryThermalMass=18.27 % Parameter assumed J/K  NumThermalModels=6 % Parameter not set  ThermalConductivityZ=18 % Parameter not set W/(K*m)  CrossSectionalAreaXY=0.000228 m^2  Height=0.0401 m  ReversibleHeatModel=simscape.battery.enum.cells.ReversibleHeatModel.Disabled  EntropicCoefficient=[0, 0, 0, 0, 0, 0, 0] % Parameter not set mV/K  CurrentDirectionality=simscape.battery.enum.cells.BatteryEnable.Disabled  stateOfCharge_specify=on  stateOfCharge_priority=High  stateOfCharge=0  stateOfCharge_nominal_specify=off  stateOfCharge_nominal_value=1  stateOfCharge_nominal_unit=1  batteryVoltage_specify=off  batteryVoltage_priority=None  batteryVoltage=0 V  batteryVoltage_nominal_specify=off  batteryVoltage_nominal_value=1  batteryVoltage_nominal_unit=V  batteryCurrent_specify=off  batteryCurrent_priority=None  batteryCurrent=0 A  batteryCurrent_nominal_specify=off  batteryCurrent_nominal_value=1  batteryCurrent_nominal_unit=A  numCycles_specify=off  numCycles_priority=High  numCycles=0  numCycles_nominal_specify=off  numCycles_nominal_value=1  numCycles_nominal_unit=1  batteryTemperature_specify=off  batteryTemperature_priority=High  batteryTemperature=298.15 K  batteryTemperature_nominal_specify=off  batteryTemperature_nominal_value=1  batteryTemperature_nominal_unit=K  hysteresisState_specify=off  hysteresisState_priority=High  hysteresisState=0  hysteresisState_nominal_specify=off  hysteresisState_nominal_value=1  hysteresisState_nominal_unit=1  isExothermFaulted_specify=off  isExothermFaulted_priority=None  isExothermFaulted=0  isExothermFaulted_nominal_specify=off  isExothermFaulted_nominal_value=1  isExothermFaulted_nominal_unit=1  reactionHeatRate_specify=off  reactionHeatRate_priority=None  reactionHeatRate=0 W  reactionHeatRate_nominal_specify=off  reactionHeatRate_nominal_value=1  reactionHeatRate_nominal_unit=W  reactionExtent_specify=off  reactionExtent_priority=None  reactionExtent=0  reactionExtent_nominal_specify=off  reactionExtent_nominal_value=1  reactionExtent_nominal_unit=1
      settings: AttributesFormatString=Panasonic:NCA673440
  Charger : batt_lib/Cyclers/Charger  charging_current=1.236 A  voltage_threshold=4.1 V  charging_voltage=4.1 V  current_threshold=0.01 A
  Compare To Constant : simulink/Logic and Bit Operations/Compare To Constant  relop=<  const=0  OutDataTypeStr=boolean
  Compare To Constant1 : simulink/Logic and Bit Operations/Compare To Constant  relop=>  const=1  OutDataTypeStr=boolean
  Convective Heat Transfer : fl_lib/Thermal/Thermal Elements/Convective Heat Transfer  thermal_type=foundation.enum.constant_variable.constant  area=0.001 m^2  heat_tr_coeff=20 W/(K*m^2)  min_heat_tr_coeff=1e-3 W/(K*m^2)  T_specify=off  T_priority=None  T=0 K  T_nominal_specify=off  T_nominal_value=1  T_nominal_unit=K  Q_specify=off  Q_priority=None  Q=0 W  Q_nominal_specify=off  Q_nominal_value=1  Q_nominal_unit=W
  Electrical Reference : fl_lib/Electrical/Electrical Elements/Electrical Reference
  PS Constant : fl_lib/Physical Signals/Sources/PS Constant  constant=1
  Probe : SimscapeProbe  BoundBlock=1  Variables="{\"batteryCurrent\":{\"Probing\":\"ON\"},\"batteryTemperature\":{\"Probing\":\"ON\"},\"batteryVoltage\":{\"Probing\":\"ON\"},\"stateOfCharge\":{\"Probing\":\"ON\"}}"
  Scope : Scope  NumInputPorts=4
      settings: ActiveDisplayYMinimum=-0.15449999999999997  ActiveDisplayYMaximum=1.3905
  Solver Configuration : nesl_utility/Solver Configuration  PhysicalDomain=network_engine_domain  SubClassName=solver  LeftPortType=input  RightPortType=generic  Tones=[]  Harmonics=[]  SimulateNoise=off  Profile=off  UseLocalSampling=off  EnableSwitchedLinearOptims=on  FrequencyDomain=off  UseCCode=off  RelTol=0.001  AbsTol=0.001  MinStep=1e-09  ToWorkspace=off  RevertToSquareIcSolve=off  NumHomotopyIterations=100  PhasorMode=off  PhasorModeNumHarmonics=1  ConsistencySolver=NEWTON_XTOL_AFTER_FTOL  CanonicalOrdering=UNORDERED  OptimizeIntermediates=UNOPTIMIZED  IndexReductionMethod=DerivativeReplacement  DoDC=off  ResidualTolerance=1e-09  ConsistencyTolSource=GLOBAL  ConsistencyAbsTol=0.001  ConsistencyRelTol=0.001  ConsistencyTolFactor=0.001  UseLocalSolver=off  LocalSolverChoice=NE_BACKWARD_EULER_ADVANCER  ResolveIndetEquations=on  FunctionEvalNumThread=1  LocalSolverSampleTime=0.001  DoFixedCost=off  MaxNonlinIter=3  MaxModeIter=2  ComputeImpulses=off  ImpulseIterations=2  LinearAlgebra=auto  LinearAlgebraNumThread=0  EquationFormulation=NE_TIME_EF  DelaysMemoryBudget=1024  AutomaticFiltering=on  FilteringTimeConstant=0.001  PartitionStorageMethod=AS_NEEDED  PartitionMemoryBudget=1024  PartitionMethod=ROBUST  MultibodyUseLocalSolver=off  MultibodyLocalSolverChoice=ODE1  MultibodyLocalSolverSampleTime=0.001
  Stop Simulation : Stop
  Stop Simulation1 : Stop
  Temperature Source : fl_lib/Thermal/Thermal Sources/Temperature Source  temperature=298.15 K
  wires:
  Probe/1 -> Scope/1  "current"
  Probe/2 -> Scope/2  "temperature"
  Probe/3 -> Scope/3  "voltage"
  Probe/4 -> Scope/4, Compare To Constant1/1, Compare To Constant/1  "soc"
  Compare To Constant/1 -> Stop Simulation/1
  Compare To Constant1/1 -> Stop Simulation1/1
  connections:
  Solver Configuration/RConn1 -- Charger/RConn2 -- Electrical Reference/LConn1 -- Battery Equivalent Circuit/RConn1
  Convective Heat Transfer/LConn1 -- Battery Equivalent Circuit/RConn2
  Temperature Source/LConn1 -- Convective Heat Transfer/RConn1
  Charger/RConn1 -- Battery Equivalent Circuit/LConn1
  PS Constant/RConn1 -- Charger/LConn1
